simulink model "OdeSetSol"  (R2018a)
settings: Solver=VariableStepAuto  StartTime=0.0  StopTime=10.0  FixedStep=0.1  RelTol=1e-3
values from neighbouring files (symbols this model uses):
  g = 40    [params.m]
  m = 5    [params.m]
settings Model: Creator=soutrik  LastModifiedBy=soutrik
settings CodeAppCC: StateflowObjectComments=on

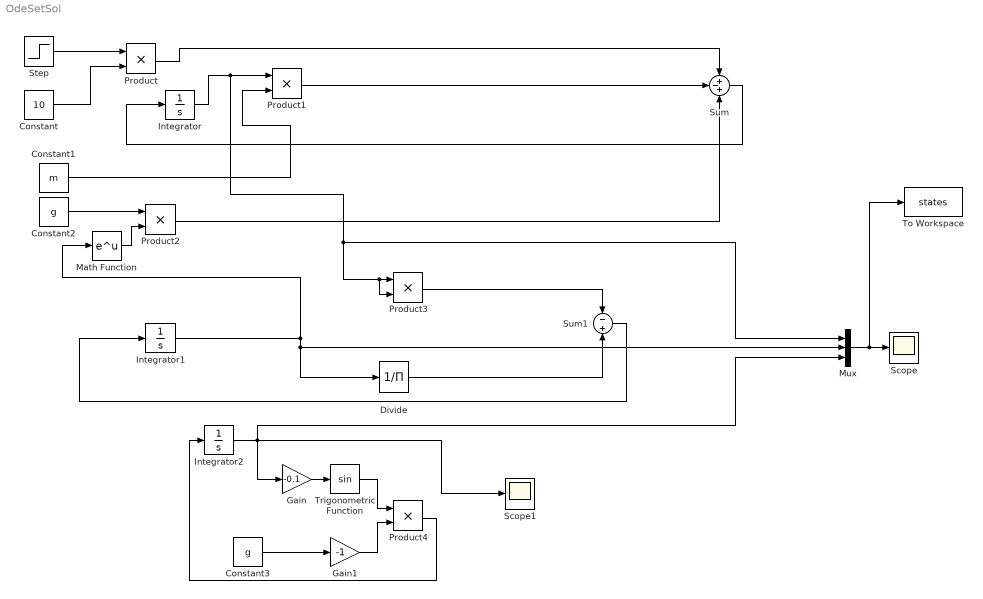
== system OdeSetSol ==
  Constant : Constant  Value=10
  Constant1 : Constant  Value=m
  Constant2 : Constant  Value=g
  Constant3 : Constant  Value=g
  Divide : Product  Inputs=/
  Gain : Gain  Gain=-0.1
  Gain1 : Gain  Gain=-1
  Integrator : Integrator  InitialCondition=3
  Integrator1 : Integrator  InitialCondition=2
  Integrator2 : Integrator  InitialCondition=-1
  Math Function : Math  SaturateOnIntegerOverflow=on
  Mux : Mux  Inputs=3
  Product{,1..4} (5 alike) : Product
  Scope : Scope
  Scope1 : Scope
  Step : Step  Time=5  SampleTime=0.1  VectorParams1D=off
  Sum : Sum  Inputs=+-+
  Sum1 : Sum  Inputs=-+
  To Workspace : ToWorkspace  VariableName=states  SampleTime=-1
  Trigonometric Function : Trigonometry
  wires:
  Step/1 -> Product/1
  Constant/1 -> Product/2
  Constant2/1 -> Product2/1
  Math Function/1 -> Product2/2
  Product/1 -> Sum/1
  Product2/1 -> Sum/3
  Sum/1 -> Integrator/1
  Constant1/1 -> Product1/2
  Product1/1 -> Sum/2
  Integrator1/1 -> Divide/1, Mux/2, Math Function/1
  Product3/1 -> Sum1/1
  Sum1/1 -> Integrator1/1
  Integrator/1 -> Mux/1, Product3/2, Product3/1, Product1/1
  Integrator2/1 -> Scope1/1, Mux/3, Gain/1
  Gain/1 -> Trigonometric Function/1
  Product4/1 -> Integrator2/1
  Gain1/1 -> Product4/2
  Trigonometric Function/1 -> Product4/1
  Constant3/1 -> Gain1/1
  Mux/1 -> To Workspace/1, Scope/1
  Divide/1 -> Sum1/2
